simulink model "loopShapingNoise"  (R2015a)
settings: Solver=ode45  StartTime=0.0  StopTime=10  RelTol=1e-3
values from neighbouring files (symbols this model uses):
  A = [0 1; 0 -c/m]    [Untitled2.m]    (also in define_consts.m; loadProperties.m; t.mat = [0  1; 0  -0.025]; test.m)
  B = [0;1/m]    [Untitled2.m]    (also in define_consts.m; loadProperties.m; t.mat = [0 0.1]; test.m = [0 0;1/m 0])
  C = [1 0]    [Untitled2.m]    (also in deadline4.m = tf([4, 1],[0, 2]); define_consts.m; loadProperties.m; t.mat)
  h_denum = 1    [LoopShaping.m]    (also in LoopShapingFilter.m = cell2mat(Hcontroller.den); LoopShapingFilterNoisy.m = cell2mat(Hcontroller.den); LoopShapingFinal.m; LoopShapingFinalCrossover.m = cell2mat(Hcontroller.den))
  h_num = 100    [LoopShaping.m]    (also in LoopShapingFilter.m = cell2mat(Hcontroller.num); LoopShapingFilterNoisy.m = cell2mat(Hcontroller.num); LoopShapingFinal.m; LoopShapingFinalCrossover.m = cell2mat(Hcontroller.num))
  s = ss(A,B,C,D)    [LoopShapingFinal.m]    (also in LoopShapingFinalCrossover.m; LoopShapingNoise.m; LoopShapingTest.m; LoopsShapingCrossover.m)
libraries: commchan3 x2, slctrlblks x1
settings Model: Creator=Adrien  LastModifiedBy=Adrien

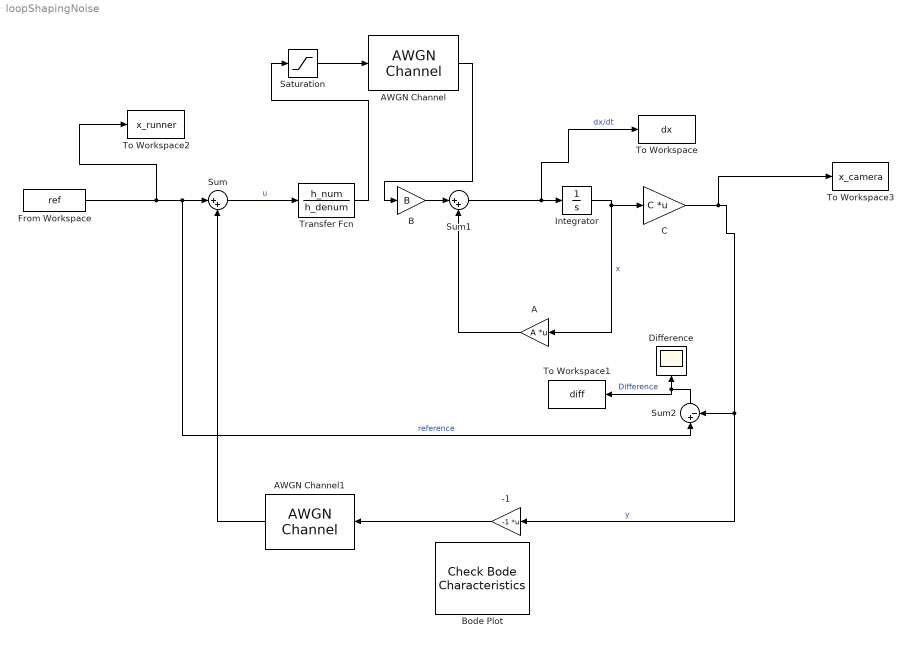
== system loopShapingNoise ==
  -1 : Gain  Gain=-1  Multiplication=Matrix(K*u) (u vector)
  A : Gain  Gain=A  Multiplication=Matrix(K*u) (u vector)
  AWGN Channel : commchan3/AWGN Channel  InputProcessing=Columns as channels (frame based)  seed=67  noiseMode=Variance from mask  EbNodB=10  EsNodB=10  SNRdB=10  bitsPerSym=1  Ps=1  Tsym=1  variance=0
  AWGN Channel1 : commchan3/AWGN Channel  InputProcessing=Columns as channels (frame based)  seed=67  noiseMode=Variance from mask  EbNodB=10  EsNodB=10  SNRdB=10  bitsPerSym=1  Ps=1  Tsym=1  variance=0.05
  "B " : Gain  Gain=B
  Bode Plot : slctrlblks/Model Verification/Check Bode  Characteristics  InstantiateOnLoad=on  SaveOperatingPoints=off  LinearizationIOs={'/Sum', 1, 'in', 'off', '';'/C ', 1, 'out', 'on', ''}  LinearizeAt=SnapshotTimes  SnapshotTimes=[0]  TriggerType=rising  SampleTime=auto  RateConversionMethod=zoh  PreWarpFreq=10  UseExactDelayModel=off  UseFullBlockNameLabels=off  UseBusSignalLabels=off  enabled=on  stopWhenAssertionFail=off  export=off  ViewDlgPos=[]  OpenViewOnLoad=off  LaunchViewOnOpen=off  FrequencyUnits=rad/s  MagnitudeUnits=dB  PhaseUnits=deg  TimeUnits=seconds  EnableUpperBound=off  UpperBoundFrequencies=[]  UpperBoundMagnitudes=[]  EnableLowerBound=off  LowerBoundFrequencies=[]  LowerBoundMagnitudes=[]
      settings: SaveToWorkspace=on
  "C " : Gain  Gain=C  Multiplication=Matrix(K*u) (u vector)
  Difference : Scope
      settings: SaveName=ScopeData2
  From Workspace : FromWorkspace  VariableName=ref  SampleTime=step  Interpolate=off  OutputAfterFinalValue=Holding final value
  Integrator : Integrator  InitialCondition=[0 0]
  Saturation : Saturate  UpperLimit=70  LowerLimit=-70
  Sum : Sum  Inputs=|++
  Sum1 : Sum  Inputs=|++
  Sum2 : Sum  Inputs=|+-
  To Workspace : ToWorkspace  VariableName=dx  SaveFormat=Timeseries  SampleTime=-1
  To Workspace1 : ToWorkspace  VariableName=diff  SaveFormat=Timeseries  SampleTime=-1
  To Workspace2 : ToWorkspace  VariableName=x_runner  SaveFormat=Timeseries  SampleTime=-1
  To Workspace3 : ToWorkspace  VariableName=x_camera  SaveFormat=Timeseries  SampleTime=-1
  Transfer Fcn : TransferFcn  Numerator=h_num  Denominator=h_denum
  wires:
  Integrator/1 -> A/1, "C "/1  "x"
  "B "/1 -> Sum1/1
  A/1 -> Sum1/2
  From Workspace/1 -> Sum/1, Sum2/1, To Workspace2/1  "reference"
  -1/1 -> AWGN Channel1/1
  "C "/1 -> To Workspace3/1, -1/1, Sum2/2  "y"
  Sum1/1 -> To Workspace/1, Integrator/1  "dx/dt"
  Sum2/1 -> To Workspace1/1, Difference/1  "Difference"
  Sum/1 -> Transfer Fcn/1  "u"
  Transfer Fcn/1 -> Saturation/1
  Saturation/1 -> AWGN Channel/1
  AWGN Channel/1 -> "B "/1
  AWGN Channel1/1 -> Sum/2
